simulink model "modeling_system_old"  (R2018a)
settings: Solver=VariableStepAuto  StartTime=0.0  StopTime=0.7  MaxStep=1e-5  RelTol=1e-3
libraries: powerlib x17, simulink x1, powerlib_meascontrol x1
settings Model: Creator=wendy  LastModifiedBy=Cyrus
settings DebuggingCC: LibraryContextMissingDiagnostic=warning

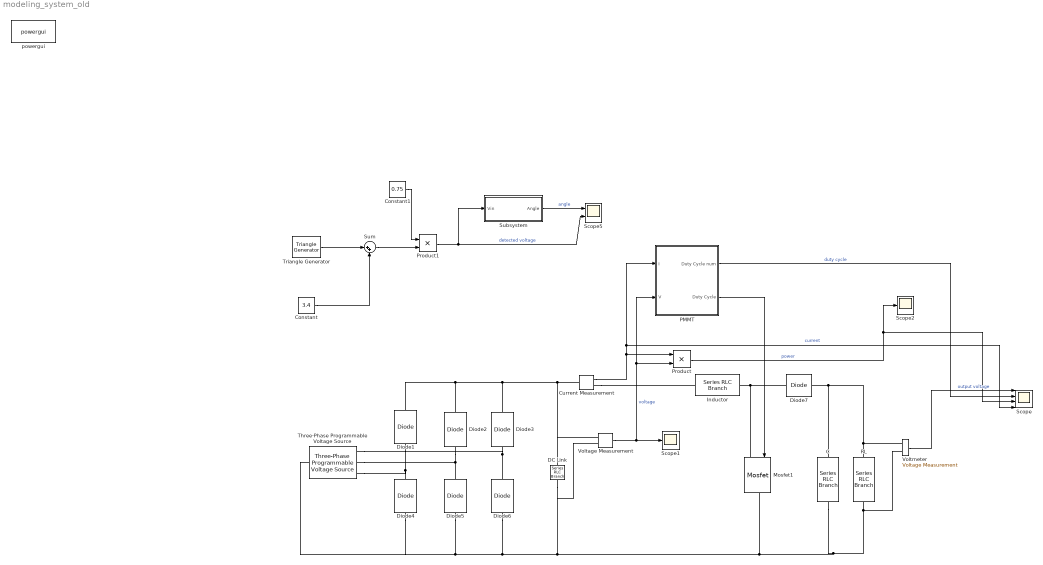
== system modeling_system_old ==
  C : powerlib/Elements/Series RLC Branch  LConnTagsString=__new0  RConnTagsString=__new0  BranchType=C  Resistance=1  Inductance=1e-3  SetiL0=off  InitialCurrent=0  Capacitance=220e-6  Setx0=off  InitialVoltage=600  Measurements=None
      settings: SourceProductName=Simscape Electrical
  Constant : Constant  Value=3.4
  Constant1 : Constant  Value=0.75
  Current Measurement : powerlib/Measurements/Current Measurement  PhasorSimulation=off  OutputType=Complex  PSBequivalent=0
      settings: SourceProductName=Simscape Electrical
  DC Link : powerlib/Elements/Series RLC Branch  LConnTagsString=__new0  RConnTagsString=__new0  BranchType=C  Resistance=1.0  Inductance=1.0  SetiL0=off  InitialCurrent=0  Capacitance=0.5  Setx0=off  InitialVoltage=310  Measurements=None
  Diode{1..6} (6 alike) : powerlib/Power Electronics/Diode  Ron=0.0001  Lon=0  Vf=0.6  IC=0  UseSnubber=off  Rs=500  Cs=250e-9  Measurements=off
  Diode7 : powerlib/Power Electronics/Diode  Ron=1e-3  Lon=0  Vf=0.6  IC=0  UseSnubber=off  Rs=inf  Cs=inf  Measurements=off
      settings: SourceProductName=Simscape Electrical
  Inductor : powerlib/Elements/Series RLC Branch  LConnTagsString=__new0  RConnTagsString=__new0  BranchType=L  Resistance=100  Inductance=500e-6  SetiL0=off  InitialCurrent=5  Capacitance=1e-6  Setx0=off  InitialVoltage=0  Measurements=None
      settings: SourceProductName=Simscape Electrical
  Mosfet1 : powerlib/Power Electronics/Mosfet  Ron=1e-3  Lon=0  Rd=1e-3  Vfd=0  IC=0  Rs=inf  Cs=inf  Measurements=off
      settings: SourceProductName=Simscape Electrical
  PMMT : Subsystem
  Product : Product
  Product1 : Product
  RL : powerlib/Elements/Series RLC Branch  LConnTagsString=__new0  RConnTagsString=__new0  BranchType=R  Resistance=30  Inductance=3e-4  SetiL0=off  InitialCurrent=5  Capacitance=1e-6  Setx0=off  InitialVoltage=0  Measurements=None
      settings: SourceProductName=Simscape Electrical
  Scope : Scope  NumInputPorts=4
  Scope1 : Scope
  Scope2 : Scope
  Scope5 : Scope  NumInputPorts=2
  Subsystem : Subsystem
  Sum : Sum  Inputs=|++
  Three-Phase Programmable Voltage Source : powerlib/Electrical Sources/Three-Phase Programmable Voltage Source  PositiveSequence=[7 0 30]  VariationEntity=None  VariationType=Table of time-amplitude pairs  VariationTypeAlt=Step  VariationStep=0.5  VariationRate=10  VariationMagnitude=0.3  VariationFrequency=2  VariationTiming=[1 2]  VariationPhaseA=off  Amplitudes=[1 0.8 1.2 1.0]  TimeValues=[0 0.1 0.15 0.2]  HarmonicGeneration=off  HarmonicA=[3 0.2 -25 0]  HarmonicB=[2 0.15 35 2]  Timing="[0.05  300]"  BusType=swing  Pref=0  Qref=0  Qmin=-inf  Qmax=inf
  Triangle Generator : powerlib_meascontrol/Pulse & Signal Generators/Triangle Generator  Freq=2  Phase=90  Ts=0
  Voltage Measurement : powerlib/Measurements/Voltage Measurement  PhasorSimulation=off  OutputType=Complex  PSBequivalent=0
      settings: SourceProductName=Simscape Electrical
  Voltmeter : powerlib/Measurements/Voltage Measurement  PhasorSimulation=off  OutputType=Complex  PSBequivalent=0
      settings: SourceProductName=Simscape Electrical
  powergui : powerlib/powergui  Priority=1  SimulationMode=Continuous  SampleTime=50e-6  frequency=60  Iterations=50  frequencyindice=0  Pbase=100e6  ErrMax=1e-4  UnitsV=kV  UnitsW=MW  buscounter=0  FunctionMessages=off  echomessages=off  EnableUseOfTLC=off  CurrentSourceSwitches=off  DisableSnubberDevices=off  DisableRonSwitches=off  DisableVfSwitches=off  DisplayEquations=off  SolverType=Tustin/Backward Euler (TBE)  Interpol=off  ExternalGateDelay=off  methode=off  Ts=100  x0status=blocks  SPID=on  SwTol=0  HookPort=off  RestoreLinks=warning  ResistiveCurrentMeasurement=off  Frange=[0:2:500]  Ylog=off  Xlog=on  ShowGrid=off  save=off  variable=ZData  structure=0  ZoomFFT=off  StartTime=0.0  cycles=1  DisplayStyle=1  fundamental=60  FreqAxis=off  MaxFrequency=1000  frequencyindicesteady=1  RmsSteady=1  display=off
  wires:
  Voltmeter/1 -> Scope/1  "output voltage"
  PMMT/2(Duty Cycle) -> Mosfet1/1
  Current Measurement/1 -> Product/1, PMMT/1(I), Scope/4  "current"
  PMMT/1(Duty Cycle num) -> Scope/2  "duty cycle"
  Voltage Measurement/1 -> PMMT/2(V), Product/2, Scope1/1  "voltage"
  Product/1 -> Scope2/1, Scope/3  "power"
  Sum/1 -> Product1/2
  Triangle Generator/1 -> Sum/1
  Constant/1 -> Sum/2
  Constant1/1 -> Product1/1
  Product1/1 -> Subsystem/1(Vin), Scope5/2  "detected voltage"
  Subsystem/1(Angle) -> Scope5/1  "angle"
  connections:
  RL/LConn1 -- C/LConn1 -- Diode7/RConn1 -- Voltmeter/LConn1
  Diode7/LConn1 -- Mosfet1/LConn1 -- Inductor/RConn1
  Current Measurement/RConn1 -- Inductor/LConn1
  Three-Phase Programmable Voltage Source/RConn1 -- Diode6/RConn1 -- Diode3/LConn1
  Three-Phase Programmable Voltage Source/RConn2 -- Diode5/RConn1 -- Diode2/LConn1
  Three-Phase Programmable Voltage Source/RConn3 -- Diode4/RConn1 -- Diode1/LConn1
  Diode2/RConn1 -- DC Link/LConn1 -- Voltage Measurement/LConn1 -- Current Measurement/LConn1 -- Diode3/RConn1 -- Diode1/RConn1
  C/RConn1 -- RL/RConn1 -- Voltmeter/LConn2 -- DC Link/RConn1 -- Voltage Measurement/LConn2 -- Diode4/LConn1 -- Three-Phase Programmable Voltage Source/LConn1 -- Diode5/LConn1 -- Diode6/LConn1 -- Mosfet1/RConn1

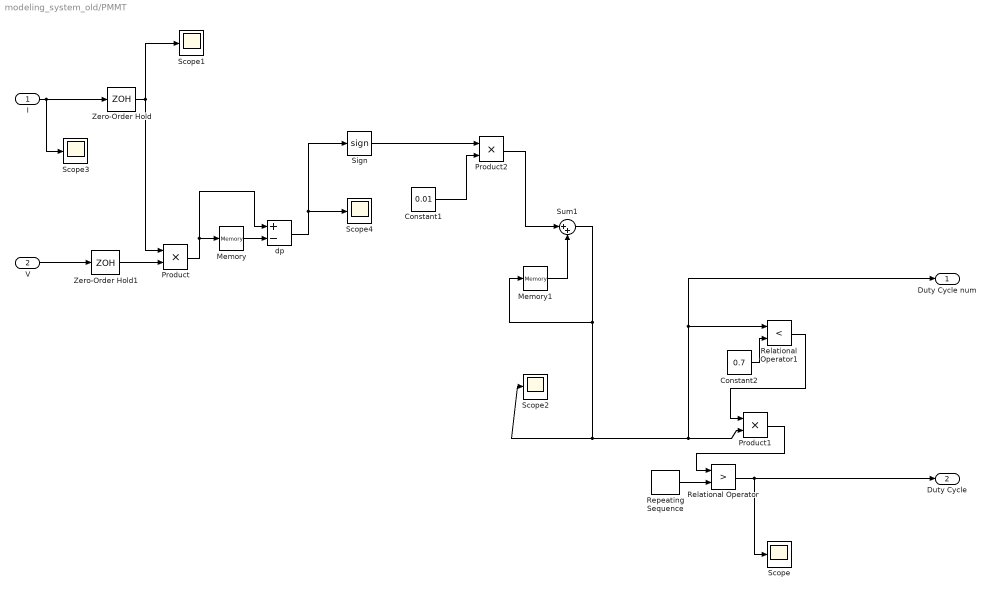
== system modeling_system_old/PMMT ==
  I : Inport
  V : Inport  Port=2
  Constant1 : Constant  Value=0.01
  Constant2 : Constant  Value=0.7
  Memory : Memory  InitialCondition=100  InheritSampleTime=on
  Memory1 : Memory  InitialCondition=0.5  InheritSampleTime=on
  Product : Product
  Product1 : Product
  Product2 : Product
  Relational Operator : RelationalOperator  Operator=>  OutDataTypeStr=boolean  RndMeth=Simplest
  Relational Operator1 : RelationalOperator  Operator=<  OutDataTypeStr=boolean  RndMeth=Simplest
  Repeating Sequence : simulink/Sources/Repeating Sequence  rep_seq_t=[0 0.00005]  rep_seq_y=[0 1]
  Scope{,1..4} (5 alike) : Scope
  Sign : Signum
  Sum1 : Sum  Inputs=|++
  Zero-Order Hold : ZeroOrderHold  SampleTime=0.06
  Zero-Order Hold1 : ZeroOrderHold  SampleTime=0.06
  dp : Sum  Inputs=+-
  Duty Cycle num : Outport
  Duty Cycle : Outport  Port=2
  wires:
  Memory/1 -> dp/2
  I/1 -> Scope3/1, Zero-Order Hold/1
  dp/1 -> Scope4/1, Sign/1
  Repeating Sequence/1 -> Relational Operator/2
  Sum1/1 -> Scope2/1, Relational Operator1/1, Duty Cycle num/1, Product1/2, Memory1/1
  Zero-Order Hold/1 -> Scope1/1, Product/1
  Sign/1 -> Product2/1
  Relational Operator/1 -> Scope/1, Duty Cycle/1
  Product2/1 -> Sum1/1
  Constant1/1 -> Product2/2
  Memory1/1 -> Sum1/2
  V/1 -> Zero-Order Hold1/1
  Zero-Order Hold1/1 -> Product/2
  Product/1 -> dp/1, Memory/1
  Constant2/1 -> Relational Operator1/2
  Relational Operator1/1 -> Product1/1
  Product1/1 -> Relational Operator/1

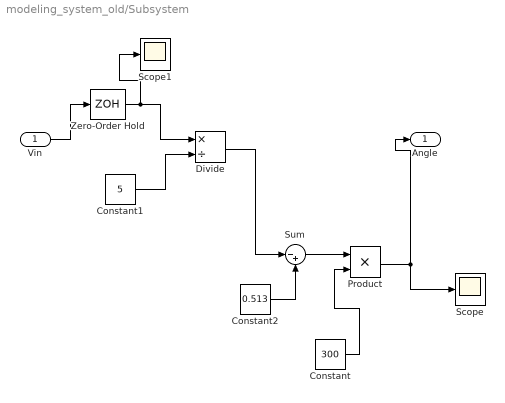
== system modeling_system_old/Subsystem ==
  Vin : Inport
  Constant : Constant  Value=300
  Constant1 : Constant  Value=5
  Constant2 : Constant  Value=0.513
  Divide : Product  Inputs=*/
  Product : Product
  Scope : Scope
  Scope1 : Scope
  Sum : Sum  Inputs=|-+
  Zero-Order Hold : ZeroOrderHold  SampleTime=0.01
  Angle : Outport
  wires:
  Constant2/1 -> Sum/2
  Sum/1 -> Product/1
  Constant/1 -> Product/2
  Product/1 -> Scope/1, Angle/1
  Divide/1 -> Sum/1
  Constant1/1 -> Divide/2
  Vin/1 -> Zero-Order Hold/1
  Zero-Order Hold/1 -> Scope1/1, Divide/1
